simulink model "Longitudinal_Dynamics_2Track"  (R2020a)
settings: Solver=VariableStepAuto  StartTime=0.0  StopTime=10.0  RelTol=1e-3
PreLoadFcn:
  | data=xlsread('spark dip analysis','spark dip analysis');
  | breakpoints1=data(2:end,1);
  | table_data=data(2:end,3);
settings Model: Creator=yafta  LastModifiedBy=Matthew

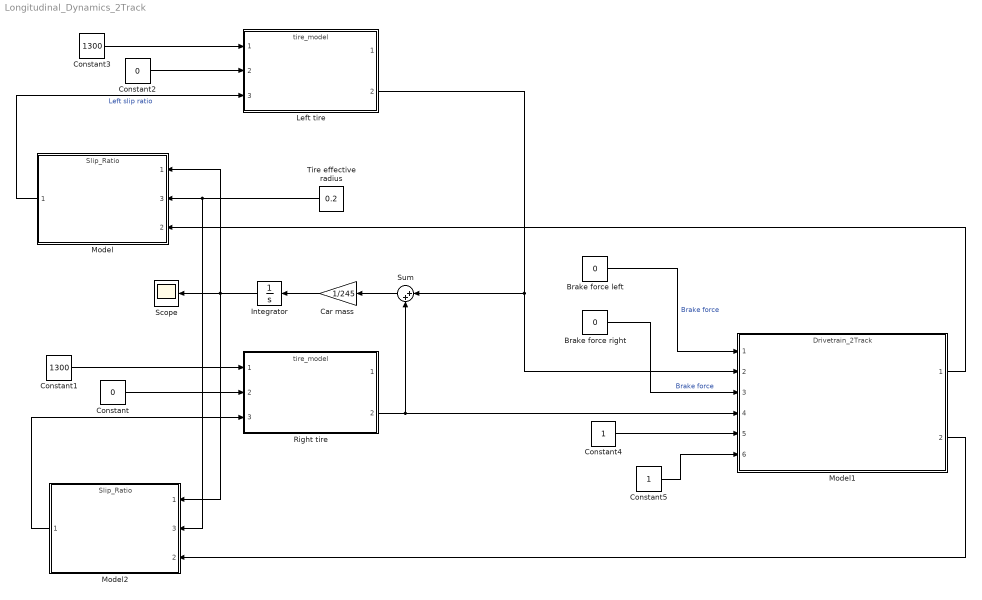
== system Longitudinal_Dynamics_2Track ==
  Brake force left : Constant  Value=0
  Brake force right : Constant  Value=0
  Car mass : Gain  Gain=1/245
  Constant : Constant  Value=0
  Constant1 : Constant  Value=1300
  Constant2 : Constant  Value=0
  Constant3 : Constant  Value=1300
  Constant4 : Constant
  Constant5 : Constant
  Integrator : Integrator  InitialCondition=25
  Left tire : ModelReference  ModelNameDialog=tire_model.slx  SimulationMode=Normal  ModelReferenceVersion=1.19
  Model : ModelReference  ModelNameDialog=Slip_Ratio  SimulationMode=Normal  ModelReferenceVersion=1.3
      settings: PortSchema="{\"entries\":[{\"content\":{\"sides\":[{\"content\":{\"connectorIds\":[\"In1\",\"In3\",\"In2\"]},\"type\":\"ConnectorPlacement.EquallySpacedRectSide\",\"uuid\":\"453251a7-84d3-4aba-8a5f-919745f4e8d1\"},{\"content\":{\"connectorIds\":[\"Out1\"],\"side\":\"RIGHT\"},\"type\":\"ConnectorPlacement.EquallySpacedRectSide\",\"uuid\":\"59fcb72d-695f-4f2f-a2f8-44c50943ff36\"},{\"content\":{\"connectorIds\":[],\"side\":\"TOP\"},\"type\":\"ConnectorPlacement.EquallySpacedRectSide\",\"uuid\":\"5a18c94f-eba1-41af-a901-0bec6681761f\"}]},\"type\":\"ConnectorPlacement.EquallySpacedConnector\",\"uuid\":\"c383bd47-7cf2-468f-9e3b-8c9d12b335a2\"}],\"packageUris\":[\"http://schema.mathworks.com/mf0/Connector/19700101\"],\"version\":\"1.0\"}"
  Model1 : ModelReference  ModelNameDialog=Drivetrain_2Track.slx  SimulationMode=Normal  ModelReferenceVersion=1.11
  Model2 : ModelReference  ModelNameDialog=Slip_Ratio  SimulationMode=Normal  ModelReferenceVersion=1.3
      settings: PortSchema="{\"entries\":[{\"content\":{\"sides\":[{\"content\":{\"connectorIds\":[\"In1\",\"In3\",\"In2\"]},\"type\":\"ConnectorPlacement.EquallySpacedRectSide\",\"uuid\":\"453251a7-84d3-4aba-8a5f-919745f4e8d1\"},{\"content\":{\"connectorIds\":[\"Out1\"],\"side\":\"RIGHT\"},\"type\":\"ConnectorPlacement.EquallySpacedRectSide\",\"uuid\":\"59fcb72d-695f-4f2f-a2f8-44c50943ff36\"},{\"content\":{\"connectorIds\":[],\"side\":\"TOP\"},\"type\":\"ConnectorPlacement.EquallySpacedRectSide\",\"uuid\":\"5a18c94f-eba1-41af-a901-0bec6681761f\"}]},\"type\":\"ConnectorPlacement.EquallySpacedConnector\",\"uuid\":\"c383bd47-7cf2-468f-9e3b-8c9d12b335a2\"}],\"packageUris\":[\"http://schema.mathworks.com/mf0/Connector/19700101\"],\"version\":\"1.0\"}"
  Right tire : ModelReference  ModelNameDialog=tire_model.slx  SimulationMode=Normal  ModelReferenceVersion=1.19
  Scope : Scope
  Sum : Sum  Inputs=|++
  Tire effective radius : Constant  Value=0.2
  wires:
  Constant1/1 -> Right tire/1
  Right tire/2 -> Sum/2, Model1/4
  Brake force right/1 -> Model1/3  "Brake force"
  Model1/2 -> Model2/2
  Model2/1 -> Right tire/3
  Constant/1 -> Right tire/2
  Constant2/1 -> Left tire/2
  Model/1 -> Left tire/3  "Left slip ratio"
  Brake force left/1 -> Model1/1  "Brake force"
  Constant3/1 -> Left tire/1
  Left tire/2 -> Sum/1, Model1/2
  Model1/1 -> Model/2
  Sum/1 -> Car mass/1
  Car mass/1 -> Integrator/1
  Integrator/1 -> Model2/1, Scope/1, Model/1
  Constant4/1 -> Model1/5
  Tire effective radius/1 -> Model2/3, Model/3
  Constant5/1 -> Model1/6
